simulink model "drone_mpc_simulink"  (R2023b)
settings: Solver=FixedStepAuto  StartTime=0.0  StopTime=end_time  RelTol=1e-3
values from neighbouring files (symbols this model uses):
  T_MPC = 0.1    [drone_mpc.m]    (also in drone_mpc_generation_following.m; drone_sfunction.m = 0.5)
settings Model: Creator=MY  LastModifiedBy=MY

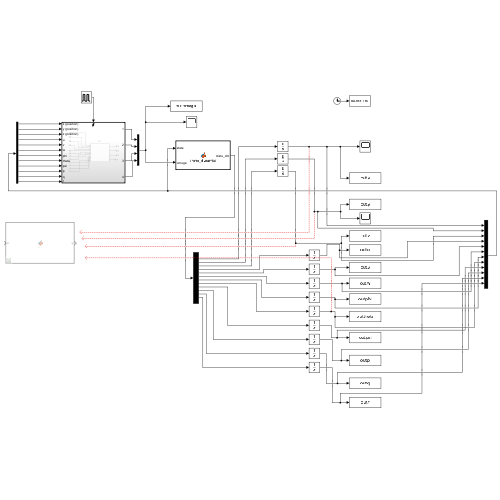
[thumbnail: Simulink's stored preview of the top-level diagram]
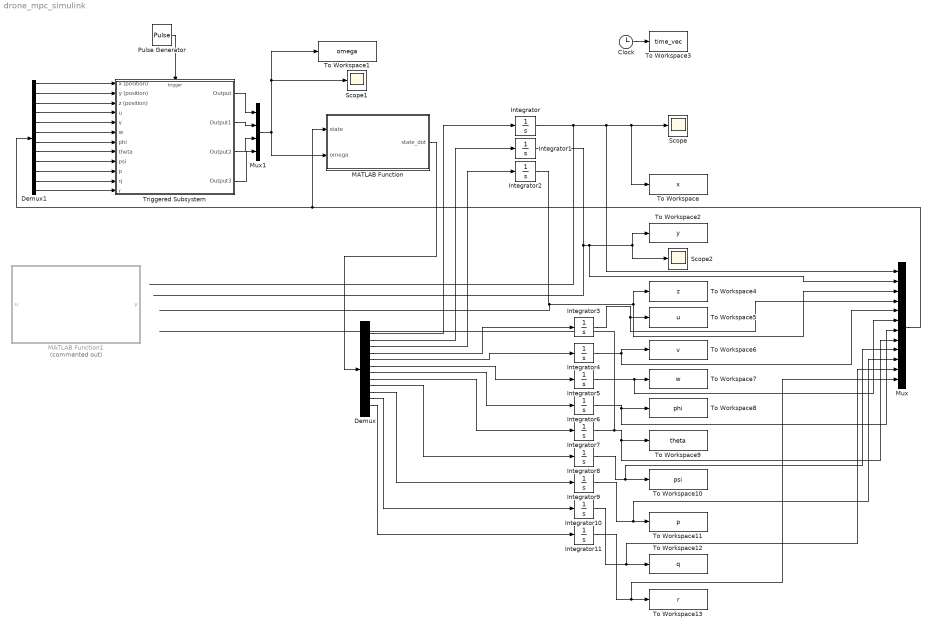
== system drone_mpc_simulink ==
  Clock : Clock
  Demux : Demux  Outputs=12
  Demux1 : Demux  Outputs=12
  Integrator{,1..11} (12 alike) : Integrator
  MATLAB Function : MATLAB Function  TreatAsAtomicUnit=on
  MATLAB Function1 : MATLAB Function  Commented=on  TreatAsAtomicUnit=on
  Mux : Mux  Inputs=12
  Mux1 : Mux
  Pulse Generator : DiscretePulseGenerator  PulseType=Time based  Period=T_MPC  PulseWidth=5
  Scope : Scope
  Scope1 : Scope
  Scope2 : Scope
  To Workspace : ToWorkspace  VariableName=x  SampleTime=-1
      settings: Save2DSignal=2-D array (concatenate along first dimension)
  To Workspace1 : ToWorkspace  VariableName=omega  SaveFormat=Timeseries  SampleTime=-1
  To Workspace10 : ToWorkspace  VariableName=psi  SampleTime=-1
      settings: Save2DSignal=2-D array (concatenate along first dimension)
  To Workspace11 : ToWorkspace  VariableName=p  SampleTime=-1
      settings: Save2DSignal=2-D array (concatenate along first dimension)
  To Workspace12 : ToWorkspace  VariableName=q  SampleTime=-1
      settings: Save2DSignal=2-D array (concatenate along first dimension)
  To Workspace13 : ToWorkspace  VariableName=r  SampleTime=-1
      settings: Save2DSignal=2-D array (concatenate along first dimension)
  To Workspace2 : ToWorkspace  VariableName=y  SampleTime=-1
      settings: Save2DSignal=2-D array (concatenate along first dimension)
  To Workspace3 : ToWorkspace  VariableName=time_vec  SampleTime=-1
  To Workspace4 : ToWorkspace  VariableName=z  SampleTime=-1
      settings: Save2DSignal=2-D array (concatenate along first dimension)
  To Workspace5 : ToWorkspace  VariableName=u  SampleTime=-1
      settings: Save2DSignal=2-D array (concatenate along first dimension)
  To Workspace6 : ToWorkspace  VariableName=v  SampleTime=-1
      settings: Save2DSignal=2-D array (concatenate along first dimension)
  To Workspace7 : ToWorkspace  VariableName=w  SampleTime=-1
      settings: Save2DSignal=2-D array (concatenate along first dimension)
  To Workspace8 : ToWorkspace  VariableName=phi  SampleTime=-1
      settings: Save2DSignal=2-D array (concatenate along first dimension)
  To Workspace9 : ToWorkspace  VariableName=theta  SampleTime=-1
      settings: Save2DSignal=2-D array (concatenate along first dimension)
  Triggered Subsystem : Subsystem  TreatAsAtomicUnit=on
  wires:
  Integrator/1 -> Mux/1, To Workspace/1, Scope/1
  Mux1/1 -> MATLAB Function/2(omega), Scope1/1, To Workspace1/1
  Integrator1/1 -> Mux/2, To Workspace2/1, Scope2/1
  Pulse Generator/1 -> Triggered Subsystem/Trigger
  Clock/1 -> To Workspace3/1
  MATLAB Function/1(state_dot) -> Demux/1
  Demux/1 -> Integrator/1
  Demux/2 -> Integrator1/1
  Demux/3 -> Integrator2/1
  Integrator2/1 -> To Workspace4/1, Mux/3
  Demux/4 -> Integrator3/1
  Demux/5 -> Integrator4/1
  Demux/6 -> Integrator5/1
  Demux/7 -> Integrator6/1
  Demux/8 -> Integrator7/1
  Demux/9 -> Integrator8/1
  Demux/10 -> Integrator9/1
  Demux/11 -> Integrator10/1
  Demux/12 -> Integrator11/1
  Integrator3/1 -> Mux/4, To Workspace5/1
  Integrator4/1 -> Mux/5, To Workspace6/1
  Integrator5/1 -> Mux/6, To Workspace7/1
  Integrator6/1 -> Mux/7, To Workspace8/1
  Integrator7/1 -> Mux/8, To Workspace9/1
  Integrator8/1 -> Mux/9, To Workspace10/1
  Integrator9/1 -> Mux/10, To Workspace11/1
  Integrator10/1 -> Mux/11, To Workspace12/1
  Integrator11/1 -> Mux/12, To Workspace13/1
  Mux/1 -> Demux1/1, MATLAB Function/1(state)
  Demux1/1 -> Triggered Subsystem/1(x (position))
  Demux1/2 -> Triggered Subsystem/2(y (position))
  Demux1/3 -> Triggered Subsystem/3(z (position))
  Demux1/4 -> Triggered Subsystem/4(u)
  Demux1/5 -> Triggered Subsystem/5(v)
  Demux1/6 -> Triggered Subsystem/6(w)
  Demux1/7 -> Triggered Subsystem/7(phi)
  Demux1/8 -> Triggered Subsystem/8(theta)
  Demux1/9 -> Triggered Subsystem/9(psi)
  Demux1/10 -> Triggered Subsystem/10(p)
  Demux1/11 -> Triggered Subsystem/11(q)
  Demux1/12 -> Triggered Subsystem/12(r)
  Triggered Subsystem/1(Output) -> Mux1/1
  Triggered Subsystem/2(Output1) -> Mux1/2
  Triggered Subsystem/3(Output2) -> Mux1/3
  Triggered Subsystem/4(Output3) -> Mux1/4

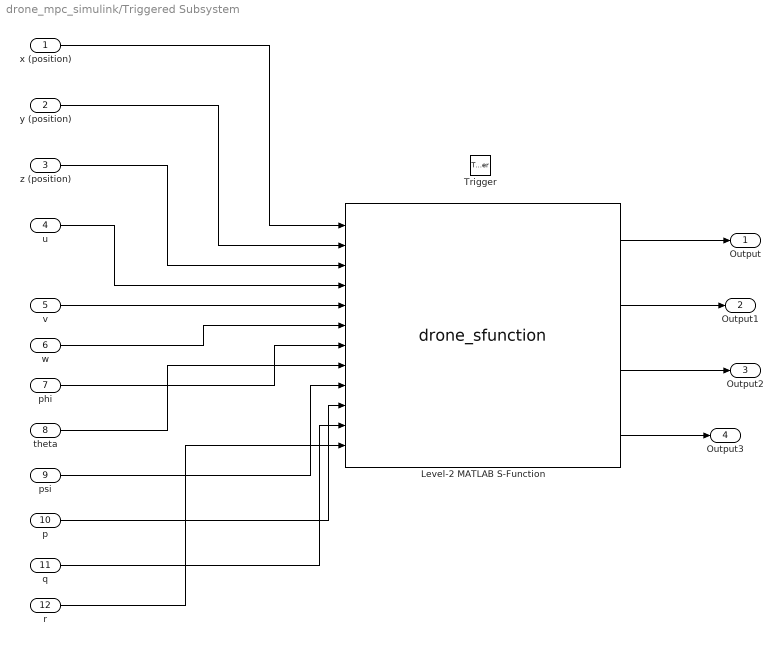
== system drone_mpc_simulink/Triggered Subsystem ==
  x (position) : Inport
  y (position) : Inport  Port=2
  z (position) : Inport  Port=3
  u : Inport  Port=4
  v : Inport  Port=5
  w : Inport  Port=6
  phi : Inport  Port=7
  theta : Inport  Port=8
  psi : Inport  Port=9
  p : Inport  Port=10
  q : Inport  Port=11
  r : Inport  Port=12
  Trigger : TriggerPort  VariantControl=(inherit)
  Level-2 MATLAB S-Function : M-S-Function  FunctionName=drone_sfunction
  Output : Outport
  Output1 : Outport  Port=2
  Output2 : Outport  Port=3
  Output3 : Outport  Port=4
  wires:
  x (position)/1 -> Level-2 MATLAB S-Function/1
  y (position)/1 -> Level-2 MATLAB S-Function/2
  z (position)/1 -> Level-2 MATLAB S-Function/3
  u/1 -> Level-2 MATLAB S-Function/4
  v/1 -> Level-2 MATLAB S-Function/5
  w/1 -> Level-2 MATLAB S-Function/6
  phi/1 -> Level-2 MATLAB S-Function/7
  theta/1 -> Level-2 MATLAB S-Function/8
  psi/1 -> Level-2 MATLAB S-Function/9
  p/1 -> Level-2 MATLAB S-Function/10
  q/1 -> Level-2 MATLAB S-Function/11
  r/1 -> Level-2 MATLAB S-Function/12
  Level-2 MATLAB S-Function/1 -> Output/1
  Level-2 MATLAB S-Function/2 -> Output1/1
  Level-2 MATLAB S-Function/3 -> Output2/1
  Level-2 MATLAB S-Function/4 -> Output3/1

== matlab function drone_mpc_simulink/MATLAB Function ==
  data: state input; omega input; state_dot output
function state_dot  = drone_dynamics(state,omega)
    state_dot = zeros(12,1);
    % Model Parameters 
    [m,g,Ix,Iy,Iz,l,k,b]=get_model();
    
    % State Vars
    % x, y, z           linear position in world frame
    % u, v, w           linear velocity in body frame
    % phi, theta, psi   euler angles
    % p, q, r           angular velocity in body frame
    x = state(1);   
    y = state(2);
    z = state(3);
    u = state(4);
    v = state(5);
    w = state(6);
    phi = state(7);
    theta = state(8);
    psi = state(9);
    p = state(10);
    q = state(11);
    r = state(12);
    omega1 = omega(1);
    omega2 = omega(2);
    omega3 = omega(3);
    omega4 = omega(4);
    
    % System inputs
    F = k*(omega1^2 + omega2^2 + omega3^2 + omega4^2);  % Total thrust (force in z body)
    tau_phi = k*l*(-omega2^2+omega4^2);                  % Torque (x body) 
    tau_theta = k*l*(omega3^2-omega1^2);                % Torque (y body)
    tau_psi = b*(-omega1^2+omega2^2-omega3^2+omega4^2);  % Torque (z body)
    
    % Translational Kinematics
    Rb2w = get_rotation_zyx(phi,theta,psi);     % Compute rotation matrix from body
    lin_vel_world = Rb2w*[u v w]';              % frame to world frame
    
    % Translational Dynamics (body frame)
    udot = r*v-q*w + g*sin(theta);
    vdot = p*w-r*u - g*cos(theta)*sin(phi);
    wdot = q*u-p*v - g*cos(theta)*cos(phi) + F/m; % account for non-inertial frame, gravity and thrust
    
    %Rotational Kinematics
    Tb2e = [1  sin(phi)*tan(theta)  cos(phi)*tan(theta);    % Compute transformation matrix from 
            0     cos(phi)               -sin(phi);         % body frame to euler angle derivatives 
            0  sin(phi)*sec(theta)  cos(phi)*sec(theta)];  
    angular_vel = Tb2e*[p q r]';
    
    % Rotational Dynamics (body frame)
    pdot = ((Iy - Iz)/Ix)*q*r + tau_phi/Ix;
    qdot = ((Iz - Ix)/Iy)*p*r + tau_theta/Iy;
    rdot = ((Ix - Iy)/Iz)*p*q + tau_psi/Iz;
    
    
    state_dot(1) = lin_vel_world(1);
    state_dot(2) = lin_vel_world(2);
    state_dot(3) = lin_vel_world(3);
    state_dot(4) = udot;
    state_dot(5) = vdot;
    state_dot(6) = wdot;
    state_dot(7) = angular_vel(1);
    state_dot(8) = angular_vel(2);
    state_dot(9) = angular_vel(3);
    state_dot(10) = pdot;
    state_dot(11) = qdot;
    state_dot(12) = rdot;

return

== matlab function drone_mpc_simulink/MATLAB Function1 ==
  data: u input; y output
function y = fcn(u)

y = u;
